simulink model "to_tank_system_2"  (R2015a)
settings: Solver=ode1  StartTime=0.0  StopTime=30.0  FixedStep=0.01  RelTol=1e-3
values from neighbouring files (symbols this model uses):
  A_1 = 5    [main.m]
  A_2 = 5    [main.m]
  k_2 = 5    [main.m]
  k_3 = 2    [main.m]
  ro = 1    [main.m]
  w_1 = 7    [main.m]
settings Model: Creator=Sondre  LastModifiedBy=Sondre

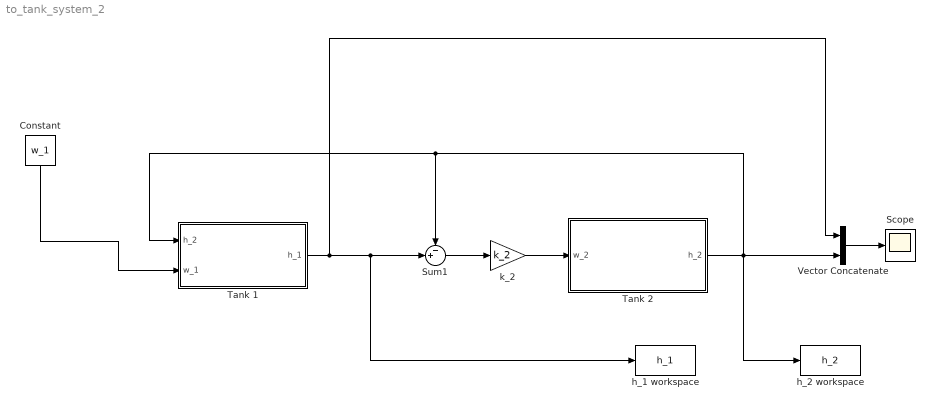
== system to_tank_system_2 ==
  Constant : Constant  Value=w_1
  Scope : Scope
  Sum1 : Sum  Inputs=-+|
  Tank 1 : Subsystem
  Tank 2 : Subsystem
  Vector Concatenate : Concatenate
  h_1 workspace : ToWorkspace  VariableName=h_1  SaveFormat=Timeseries  SampleTime=-1
  h_2 workspace : ToWorkspace  VariableName=h_2  SaveFormat=Timeseries  SampleTime=-1
  k_2 : Gain  Gain=k_2
  wires:
  Tank 2/1(h_2) -> Tank 1/1(h_2), Sum1/1, h_2 workspace/1, Vector Concatenate/2
  Sum1/1 -> k_2/1
  k_2/1 -> Tank 2/1(w_2)
  Tank 1/1(h_1) -> Vector Concatenate/1, h_1 workspace/1, Sum1/2
  Vector Concatenate/1 -> Scope/1
  Constant/1 -> Tank 1/2(w_1)

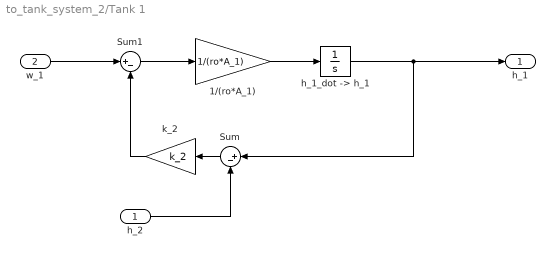
== system to_tank_system_2/Tank 1 ==
  h_2 : Inport
  w_1 : Inport  Port=2
  1/(ro*A_1) : Gain  Gain=1/(ro*A_1)
  Sum : Sum  Inputs=|+-
  Sum1 : Sum  Inputs=|+-
  "h_1_dot -> h_1" : Integrator
  k_2 : Gain  Gain=k_2
  h_1 : Outport
  wires:
  "h_1_dot -> h_1"/1 -> h_1/1, Sum/1
  Sum1/1 -> 1/(ro*A_1)/1
  h_2/1 -> Sum/2
  w_1/1 -> Sum1/1
  Sum/1 -> k_2/1
  1/(ro*A_1)/1 -> "h_1_dot -> h_1"/1
  k_2/1 -> Sum1/2

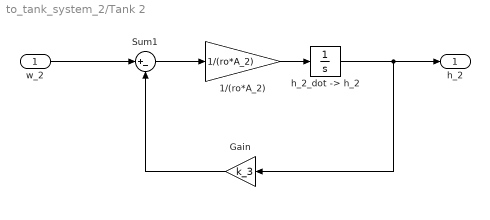
== system to_tank_system_2/Tank 2 ==
  w_2 : Inport
  1/(ro*A_2) : Gain  Gain=1/(ro*A_2)
  Gain : Gain  Gain=k_3
  Sum1 : Sum  Inputs=|+-
  "h_2_dot -> h_2" : Integrator
  h_2 : Outport
  wires:
  Gain/1 -> Sum1/2
  w_2/1 -> Sum1/1
  Sum1/1 -> 1/(ro*A_2)/1
  1/(ro*A_2)/1 -> "h_2_dot -> h_2"/1
  "h_2_dot -> h_2"/1 -> h_2/1, Gain/1
